simulink model "data_inspector_test"  (R2020a)
settings: Solver=VariableStepAuto  StartTime=0.0  StopTime=512/1e6  RelTol=1e-3
undefined symbols (not defined in the file): frame_size, fs
libraries: dspsigops x2, dspsrcs4 x2, hdlsllib x1, data_inspector x1
settings Model: Creator=LDM  LastModifiedBy=LDM
settings OptimizationCC: BlockReduction=off  ConditionallyExecuteInputs=off  DefaultParameterBehavior=Inlined
settings DebuggingCC: AlgebraicLoopMsg=error
settings HardwareCC: ProdBitPerPointer=32  ProdBitPerSizeT=32  ProdBitPerPtrDiffT=32  ProdLargestAtomicFloat=None  ProdIntDivRoundTo=Undefined  ProdEndianess=Unspecified  ProdWordSize=32  ProdHWDeviceType=ASIC/FPGA->ASIC/FPGA  TargetBitPerPointer=64  TargetBitPerSizeT=64  TargetBitPerPtrDiffT=64  TargetLongLongMode=on  TargetIntDivRoundTo=Zero  TargetEndianess=LittleEndian  TargetWordSize=64  TargetHWDeviceType=Custom Processor->MATLAB Host Computer  ProdEqTarget=off

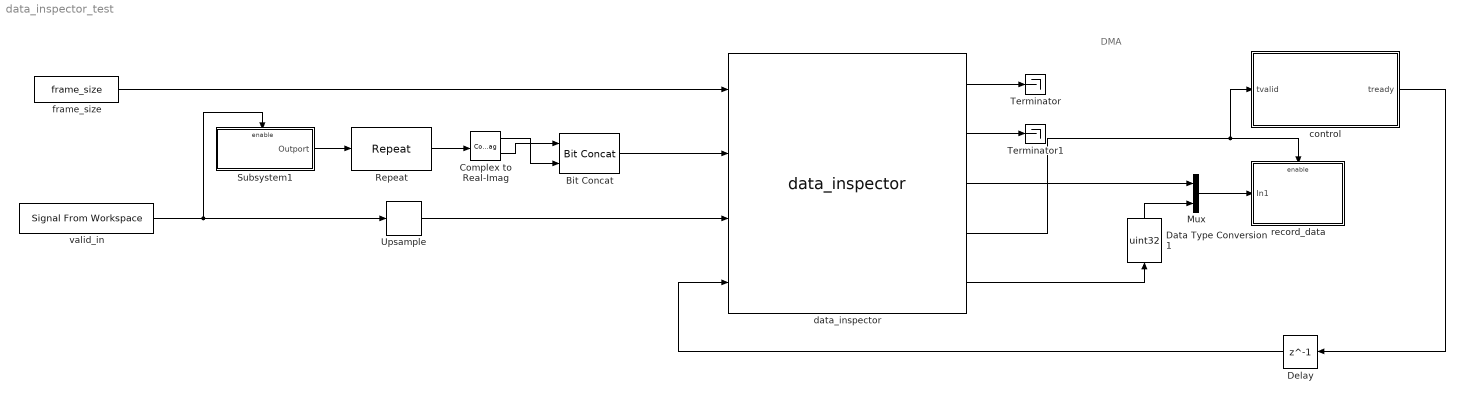
== system data_inspector_test ==
  note: DMA
  Bit Concat : hdlsllib/Logic and Bit Operations/Bit Concat  numInputs=2
  Complex to Real-Imag : ComplexToRealImag
  Data Type Conversion1 : DataTypeConversion  OutDataTypeStr=uint32
  Delay : Delay  DelayLength=1
  Mux : Mux  Inputs=2
  Repeat : dspsigops/Repeat  N=12  InputProcessing=Columns as channels (frame based)  RateOptions=Allow multirate processing  ic=0  mode=Unused parameter value
  Subsystem1 : Subsystem
  Terminator : Terminator
  Terminator1 : Terminator
  Upsample : dspsigops/Upsample  N=12  phase=0  RateOptions=Allow multirate processing  ic=0  mode=Unused parameter value
  control : Stateflow chart  TreatAsAtomicUnit=on
  data_inspector : data_inspector/data_inspector  SystemSampleTime=-1  Latency=0  AutoFrameSizeCalculation=off
  frame_size : Constant  Value=frame_size  OutDataTypeStr=uint32  SampleTime=1/(fs*12)
  record_data : Subsystem
  valid_in : dspsrcs4/Signal From Workspace  X=[true(1,randi(10)) false(1,randi(10)) true(1,randi(10))]  Ts=1/1e6  nsamps=1  OutputAfterFinalValue=Cyclic repetition  ignoreOrWarnInputAndFrameLengths=off  OutputFrames=off
  wires:
  control/1(tready) -> Delay/1
  Subsystem1/1(Outport) -> Repeat/1
  frame_size/1 -> data_inspector/1
  valid_in/1 -> Upsample/1, Subsystem1/Enable
  Repeat/1 -> Complex to Real-Imag/1
  Delay/1 -> data_inspector/4
  Mux/1 -> record_data/1(In1)
  data_inspector/3 -> Mux/1
  Complex to Real-Imag/1 -> Bit Concat/2
  Complex to Real-Imag/2 -> Bit Concat/1
  Bit Concat/1 -> data_inspector/2
  Upsample/1 -> data_inspector/3
  data_inspector/4 -> record_data/Enable, control/1(tvalid)
  data_inspector/5 -> Data Type Conversion1/1
  Data Type Conversion1/1 -> Mux/2
  data_inspector/1 -> Terminator/1
  data_inspector/2 -> Terminator1/1

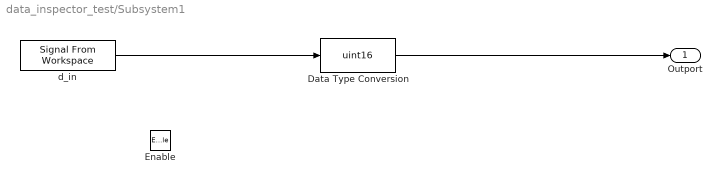
== system data_inspector_test/Subsystem1 ==
  Enable : EnablePort
  Data Type Conversion : DataTypeConversion  OutDataTypeStr=uint16
  d_in : dspsrcs4/Signal From Workspace  X=1:frame_size  Ts=1/1e6  nsamps=1  OutputAfterFinalValue=Cyclic repetition  ignoreOrWarnInputAndFrameLengths=off  OutputFrames=off
  Outport : Outport
  wires:
  d_in/1 -> Data Type Conversion/1
  Data Type Conversion/1 -> Outport/1

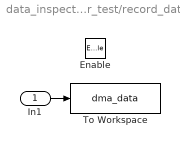
== system data_inspector_test/record_data ==
  In1 : Inport
  Enable : EnablePort
  To Workspace : ToWorkspace  VariableName=dma_data  SampleTime=-1
      settings: Save2DSignal=2-D array (concatenate along first dimension)
  wires:
  In1/1 -> To Workspace/1

== stateflow chart data_inspector_test/control ==
  state init
    % variables
    count = 0;
    d_count = 0;
  state start_frame
    %variables
    if tvalid == true
    d_count = d_count + 1
    end
    %outputs
    tready = true
  state wait
    % variables
    count = count + 1;
    %outputs
    tready = false
  state pause
    % variables
    count = count + 1;
    %outputs
    tready = false
  state end_frame
    %variables
    if tvalid == true
    d_count = d_count + 1
    end
    %outputs
    tready = true
  (default) -> init
  init -> wait
  wait -> start_frame : [count > randi(100)]{count = 0}
  end_frame -> wait : [d_count == frame_size]{d_count = 0}
  start_frame -> pause : [d_count == 3]
  pause -> end_frame : [count > randi(100)]{count = 0}
  data: tready output boolean; d_count local; count local; tvalid input; frame_size constant double =frame_size
